simulink model "time_variant_invariant_system_ex2"  (R2018b)
settings: Solver=FixedStepAuto  StartTime=0.0  StopTime=20  FixedStep=1e-3  RelTol=1e-3
settings Model: Creator=auralius  LastModifiedBy=auralius

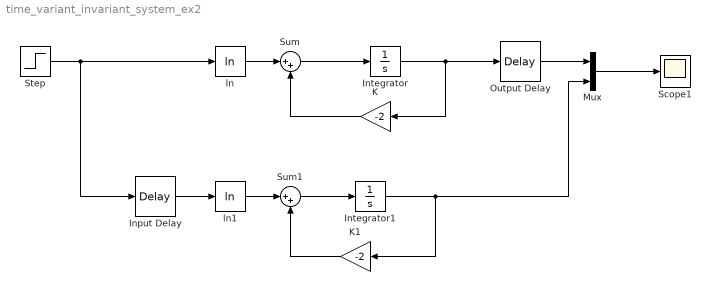
== system time_variant_invariant_system_ex2 ==
  Input Delay : TransportDelay  DelayTime=4  InitialOutput=1
  Integrator : Integrator
  Integrator1 : Integrator
  K : Gain  Gain=-2
  K1 : Gain  Gain=-2
  Mux : Mux  Inputs=2
  Output Delay : TransportDelay  DelayTime=4
  Scope1 : Scope
  Step : Step  Before=1  After=2
  Sum : Sum  Inputs=|++
  Sum1 : Sum  Inputs=|++
  ln : Math  Operator=log  SaturateOnIntegerOverflow=on
  ln1 : Math  Operator=log  SaturateOnIntegerOverflow=on
  wires:
  Integrator/1 -> K/1, Output Delay/1
  ln/1 -> Sum/1
  K/1 -> Sum/2
  Sum/1 -> Integrator/1
  Sum1/1 -> Integrator1/1
  Input Delay/1 -> ln1/1
  Integrator1/1 -> Mux/2, K1/1
  K1/1 -> Sum1/2
  ln1/1 -> Sum1/1
  Step/1 -> Input Delay/1, ln/1
  Output Delay/1 -> Mux/1
  Mux/1 -> Scope1/1
